simulink model "sig_mod_block"  (R2019a)
settings: Solver=VariableStepAuto  StartTime=0.0  StopTime=10.0  RelTol=1e-3
undefined symbols (not defined in the file): intmax, sigbuilder_block
settings Model: Creator=a3bawa  LastModifiedBy=a3bawa

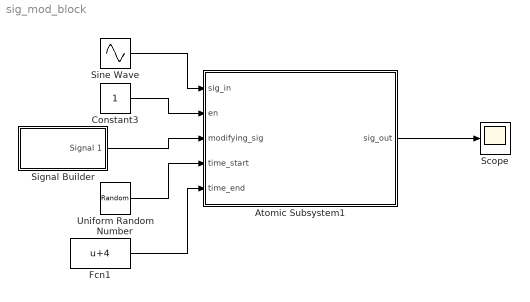
== system sig_mod_block ==
  Atomic Subsystem1 : Subsystem  TreatAsAtomicUnit=on
  Constant3 : Constant
  Fcn1 : Fcn  Expr=u+4
  Scope : Scope
  Signal Builder : Subsystem  Tag=STV Subsys  LoadFcn=sigbuilder_block('load');  StartFcn=sigbuilder_block('start');  StopFcn=sigbuilder_block('stop');  ClipboardFcn=sigbuilder_block('clipboard');  mask(Sigbuilder block){tuvar=[0:10]}
      mask help: Simulink:masks:SigbuilderBlock_MD
      mask init:
      | if ~strcmp(get_param(bdroot(gcbh),'SimulationStatus'),'stopped') tuvar = sigbuilder_block('maskInit'); end
      settings: CopyFcn=sigbuilder_block('copy');  DeleteFcn=sigbuilder_block('delete');  ModelCloseFcn=sigbuilder_block('modelClose');  PreSaveFcn=sigbuilder_block('preSave');  PauseFcn=sigbuilder_block('pause');  ContinueFcn=sigbuilder_block('continue');  NameChangeFcn=sigbuilder_block('namechange');  OpenFcn=sigbuilder_block('open',[152 61.5 550.5 362.5 ]);  CloseFcn=sigbuilder_block('close');
      mask Display: plot(0, 0, 100, 100,[2, 2, 32, 32, 2], [68, 8, 8, 68, 68],[32, 2], [38, 38], [32, 19, 2],[53, 60, 44], [32, 17, 17, 2],[16, 16, 31, 31]);txt = getActiveGroup(gcbh);text(2, 100, txt,'verticalAlignment', 'top');
  Sine Wave : Sin  SampleTime=0
  Uniform Random Number : UniformRandomNumber  Minimum=0  Maximum=6  Seed=randi(intmax)  SampleTime=0.1
  wires:
  Sine Wave/1 -> Atomic Subsystem1/1(sig_in)
  Constant3/1 -> Atomic Subsystem1/2(en)
  Signal Builder/1(Signal 1) -> Atomic Subsystem1/3(modifying_sig)
  Uniform Random Number/1 -> Atomic Subsystem1/4(time_start)
  Fcn1/1 -> Atomic Subsystem1/5(time_end)
  Atomic Subsystem1/1(sig_out) -> Scope/1

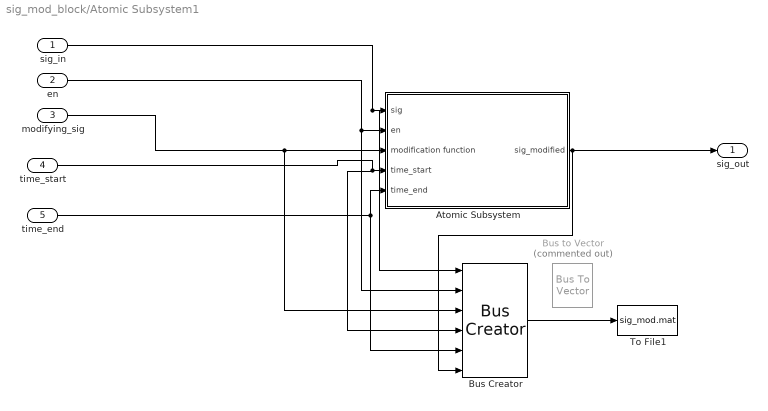
== system sig_mod_block/Atomic Subsystem1 ==
  sig_in : Inport
  en : Inport  Port=2
  modifying_sig : Inport  Port=3
  time_start : Inport  Port=4
  time_end : Inport  Port=5
  Atomic Subsystem : Subsystem  TreatAsAtomicUnit=on
  Bus Creator : BusCreator  Inputs=6
  Bus to Vector : BusToVector  Commented=on
  To File1 : ToFile  Filename=sig_mod.mat  MatrixName=signal  SaveFormat=Timeseries
  sig_out : Outport
  wires:
  time_end/1 -> Bus Creator/5, Atomic Subsystem/5(time_end)
  en/1 -> Atomic Subsystem/2(en), Bus Creator/2
  Atomic Subsystem/1(sig_modified) -> sig_out/1, Bus Creator/6
  sig_in/1 -> Bus Creator/1, Atomic Subsystem/1(sig)
  time_start/1 -> Bus Creator/4, Atomic Subsystem/4(time_start)
  modifying_sig/1 -> Atomic Subsystem/3(modification function), Bus Creator/3
  Bus Creator/1 -> To File1/1

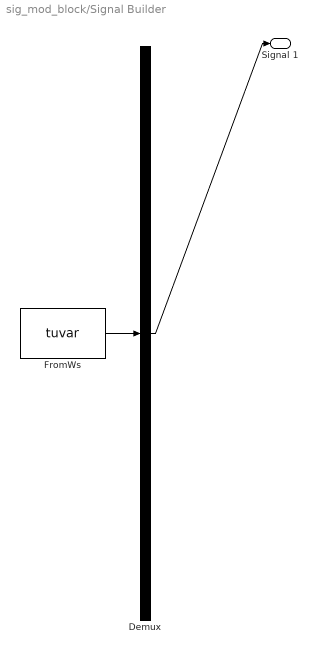
== system sig_mod_block/Signal Builder ==
  Demux : Demux  Tag=STV Demux  Outputs=1
  FromWs : FromWorkspace  Tag=STV FromWs  VariableName=tuvar  SampleTime=0
      SigBuilderData=|
      | common.afterFinalStr = 'Extrapolate'
      | common.sampleTime = 0
      | dataSet.timeRange = [0 10]
      | dataSet.name = 'Group 1'
      | sbobj.Groups.Name = 'Group 1'
      | sbobj.Groups.Signals.Name = 'Signal 1'
      | sbobj.Groups.Signals.XData = [0 1 1 2 2 3 3 4 4 5 5 6 6 7 7 8 8 9 9 10]
      | sbobj.Groups.Signals.YData = [0 0.5 0 1 0 1.5 0 2 0 1.5 0 1 0 0.5 0 1 0 1.5 0 2]
  Signal 1 : Outport  Tag=STV Outport
  wires:
  FromWs/1 -> Demux/1
  Demux/1 -> Signal 1/1

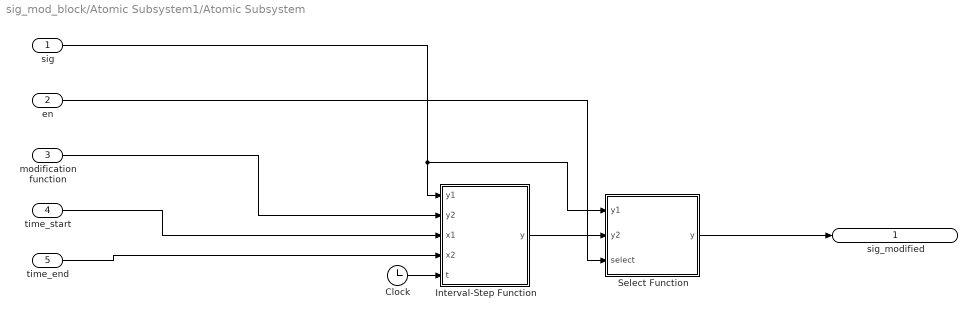
== system sig_mod_block/Atomic Subsystem1/Atomic Subsystem ==
  sig : Inport
  en : Inport  Port=2
  modification function : Inport  Port=3
  time_start : Inport  Port=4
  time_end : Inport  Port=5
  Clock : Clock
  Interval-Step Function : MATLAB Function  TreatAsAtomicUnit=on
  Select Function : MATLAB Function  TreatAsAtomicUnit=on
  sig_modified : Outport
  wires:
  Interval-Step Function/1(y) -> Select Function/2(y2)
  Clock/1 -> Interval-Step Function/5(t)
  en/1 -> Select Function/3(select)
  sig/1 -> Interval-Step Function/1(y1), Select Function/1(y1)
  Select Function/1(y) -> sig_modified/1
  modification function/1 -> Interval-Step Function/2(y2)
  time_start/1 -> Interval-Step Function/3(x1)
  time_end/1 -> Interval-Step Function/4(x2)

== matlab function sig_mod_block/Atomic Subsystem1/Atomic Subsystem/Interval-Step Function ==
  data: y1 input; y output; y2 input; x1 input; x2 input; t input
function y = fcn(y1,y2,x1,x2,t)

if (x1<=t)&&(t<x2)
    y=y2;
else
    y=y1;
end

== matlab function sig_mod_block/Atomic Subsystem1/Atomic Subsystem/Select Function ==
  data: y1 input; y output; y2 input; select input
function y = fcn(y1,y2,select)

if select>=1
    y=y2;
else
    y=y1;
end
